simulink model "Simulation"  (R2018a)
settings: Solver=VariableStepAuto  StartTime=0.0  StopTime=inf  RelTol=1e-3
libraries: powerlib x28, simulink x3, rectifier_leg x3, inverter_leg x3, powerlib_meascontrol x1
settings Model: Creator=elasfory  LastModifiedBy=AL-MOSTAFA

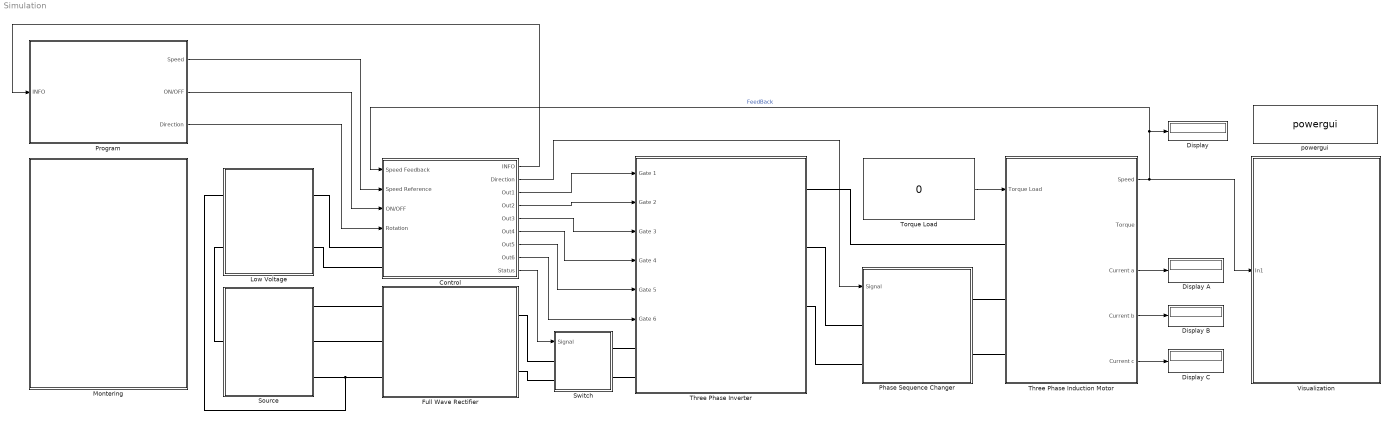
== system Simulation ==
  Control : Subsystem
  Display : Display
  Display A : Display
  Display B : Display
  Display C : Display
  Full Wave Rectifier : Subsystem
  Low Voltage : Subsystem
  Montering : Subsystem
  Phase Sequence Changer : Subsystem
  Program : Subsystem
  Source : Subsystem
  Switch : Subsystem
  Three Phase Induction Motor : Subsystem
  Three Phase Inverter : Subsystem
  Torque Load : Constant  Value=0
  Visualization : Subsystem
  powergui : powerlib/powergui  Priority=1  SimulationMode=Continuous  SampleTime=50e-6  frequency=60  Iterations=50  frequencyindice=0  Pbase=100e6  ErrMax=1e-4  UnitsV=kV  UnitsW=MW  buscounter=0  FunctionMessages=off  echomessages=off  EnableUseOfTLC=off  CurrentSourceSwitches=off  DisableSnubberDevices=off  DisableRonSwitches=off  DisableVfSwitches=off  DisplayEquations=off  SolverType=Tustin/Backward Euler (TBE)  Interpol=off  ExternalGateDelay=off  methode=off  Ts=100  x0status=blocks  SPID=on  SwTol=0  HookPort=off  RestoreLinks=warning  ResistiveCurrentMeasurement=off  Frange=[0:2:500]  Ylog=off  Xlog=on  ShowGrid=off  save=off  variable=ZData  structure=0  ZoomFFT=off  StartTime=0.0  cycles=1  DisplayStyle=1  fundamental=60  FreqAxis=off  MaxFrequency=1000  frequencyindicesteady=1  RmsSteady=1  display=off
  wires:
  Control/8(Out6) -> Three Phase Inverter/6(Gate 6)
  Control/7(Out5) -> Three Phase Inverter/5(Gate 5)
  Control/6(Out4) -> Three Phase Inverter/4(Gate 4)
  Control/5(Out3) -> Three Phase Inverter/3(Gate 3)
  Control/4(Out2) -> Three Phase Inverter/2(Gate 2)
  Control/3(Out1) -> Three Phase Inverter/1(Gate 1)
  Three Phase Induction Motor/1(Speed) -> Visualization/1(In1), Display/1, Control/1(Speed Feedback)  "FeedBack"
  Torque Load/1 -> Three Phase Induction Motor/1(Torque Load)
  Program/1(Speed) -> Control/2(Speed Reference)
  Three Phase Induction Motor/3(Current a) -> Display A/1
  Three Phase Induction Motor/4(Current b) -> Display B/1
  Three Phase Induction Motor/5(Current c) -> Display C/1
  Program/2(ON/OFF) -> Control/3(ON/OFF)
  Program/3(Direction) -> Control/4(Rotation)
  Control/9(Status) -> Switch/1(Signal)
  Control/2(Direction) -> Phase Sequence Changer/1(Signal)
  Control/1(INFO) -> Program/1(INFO)
  connections:
  Source/RConn1 -- Full Wave Rectifier/LConn1
  Source/RConn2 -- Full Wave Rectifier/LConn2
  Source/RConn3 -- Low Voltage/LConn1 -- Full Wave Rectifier/LConn3
  Three Phase Inverter/RConn1 -- Three Phase Induction Motor/LConn1
  Three Phase Inverter/RConn2 -- Phase Sequence Changer/LConn1
  Three Phase Inverter/RConn3 -- Phase Sequence Changer/LConn2
  Phase Sequence Changer/RConn1 -- Three Phase Induction Motor/LConn2
  Phase Sequence Changer/RConn2 -- Three Phase Induction Motor/LConn3
  Full Wave Rectifier/RConn1 -- Switch/LConn1
  Full Wave Rectifier/RConn2 -- Switch/LConn2
  Switch/RConn1 -- Three Phase Inverter/LConn1
  Switch/RConn2 -- Three Phase Inverter/LConn2
  Low Voltage/RConn1 -- Control/LConn1
  Low Voltage/RConn2 -- Control/LConn2
  Source/LConn1 -- Low Voltage/LConn2

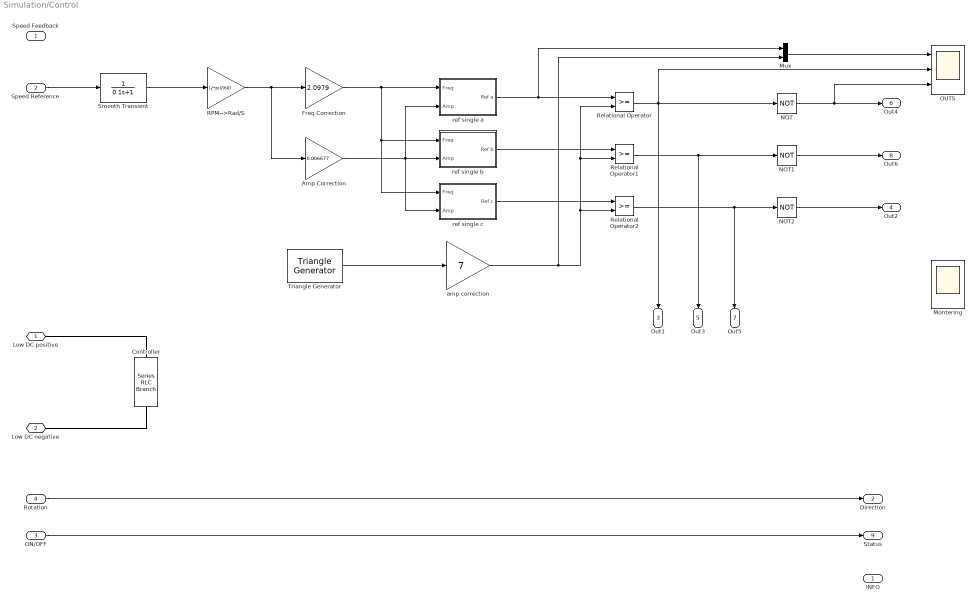
== system Simulation/Control ==
  Speed Feedback : Inport
  Speed Reference : Inport  Port=2
  ON/OFF : Inport  Port=3
  Rotation : Inport  Port=4
  Amp Correction : Gain  Gain=0.006677
  Controller : powerlib/Elements/Series RLC Branch  LConnTagsString=__new0  RConnTagsString=__new0  BranchType=R  Resistance=220  Inductance=1e-3  SetiL0=off  InitialCurrent=0  Capacitance=500*10^-6  Setx0=off  InitialVoltage=0  Measurements=None
  Freq Correction : Gain  Gain=2.0979
  Montering : Scope  NumInputPorts=2
  Mux : Mux  Inputs=2
  NOT : Logic  Operator=NOT  IconShape=distinctive  AllPortsSameDT=off  OutDataTypeStr=boolean
  NOT1 : Logic  Operator=NOT  IconShape=distinctive  AllPortsSameDT=off  OutDataTypeStr=boolean
  NOT2 : Logic  Operator=NOT  IconShape=distinctive  AllPortsSameDT=off  OutDataTypeStr=boolean
  OUTS : Scope  NumInputPorts=3
  RPM-->Rad/S : Gain  Gain=(2*pi)/(60)
  Relational Operator : RelationalOperator  OutDataTypeStr=boolean  RndMeth=Simplest
  Relational Operator1 : RelationalOperator  OutDataTypeStr=boolean  RndMeth=Simplest
  Relational Operator2 : RelationalOperator  OutDataTypeStr=boolean  RndMeth=Simplest
  Smooth Transient : TransferFcn  Denominator=[0.1 1]
  Triangle Generator : powerlib_meascontrol/Pulse & Signal Generators/Triangle Generator  Freq=1e3  Phase=90  Ts=0
  amp correction : Gain  Gain=7
  ref single a : Subsystem
  ref single b : Subsystem
  ref single c : Subsystem
  Low DC positive : PMIOPort  Side=Left
  Low DC negative : PMIOPort  Port=2  Side=Left
  INFO : Outport
  Direction : Outport  Port=2
  Out1 : Outport  Port=3
  Out2 : Outport  Port=4
  Out3 : Outport  Port=5
  Out4 : Outport  Port=6
  Out5 : Outport  Port=7
  Out6 : Outport  Port=8
  Status : Outport  Port=9
  wires:
  amp correction/1 -> Relational Operator/2, Relational Operator1/2, Relational Operator2/2, Mux/2
  ON/OFF/1 -> Status/1
  Rotation/1 -> Direction/1
  ref single a/1(Ref a) -> Mux/1, Relational Operator/1
  RPM-->Rad/S/1 -> Freq Correction/1, Amp Correction/1
  Freq Correction/1 -> ref single c/1(Freq), ref single b/1(Freq), ref single a/1(Freq)
  Amp Correction/1 -> ref single c/2(Amp), ref single a/2(Amp), ref single b/2(Amp)
  ref single b/1(Ref b) -> Relational Operator1/1
  ref single c/1(Ref c) -> Relational Operator2/1
  Relational Operator/1 -> OUTS/2, NOT/1, Out1/1
  Relational Operator1/1 -> NOT1/1, Out3/1
  Relational Operator2/1 -> NOT2/1, Out5/1
  NOT2/1 -> Out2/1
  NOT1/1 -> Out6/1
  NOT/1 -> Out4/1, OUTS/3
  Triangle Generator/1 -> amp correction/1
  Mux/1 -> OUTS/1
  Speed Reference/1 -> Smooth Transient/1
  Smooth Transient/1 -> RPM-->Rad/S/1
  connections:
  Controller/LConn1 -- Low DC positive/RConn1
  Low DC negative/RConn1 -- Controller/RConn1

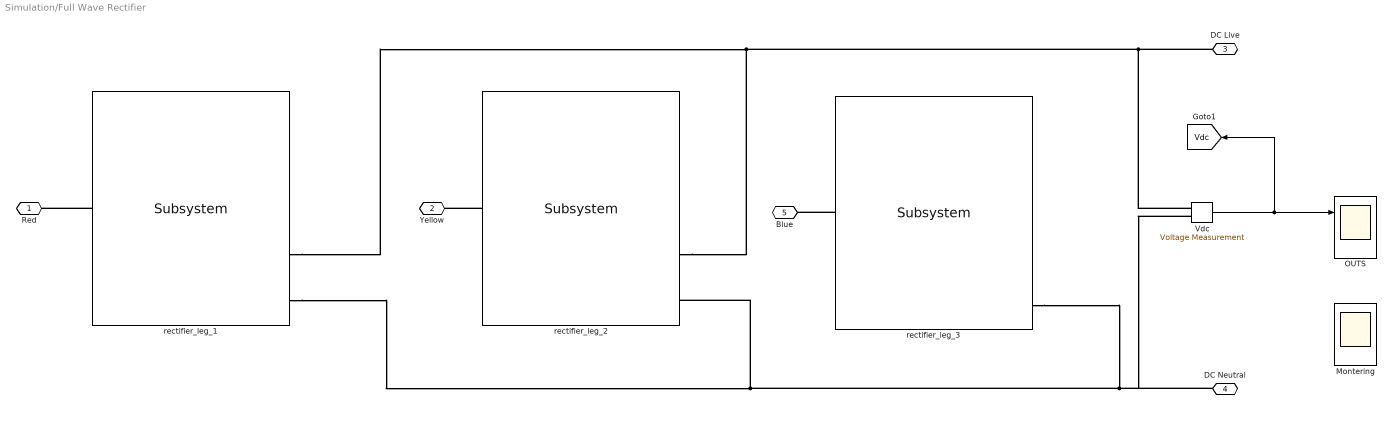
== system Simulation/Full Wave Rectifier ==
  Montering : Scope  NumInputPorts=4
  OUTS : Scope  NumInputPorts=2
  Vdc : powerlib/Measurements/Voltage Measurement  PhasorSimulation=off  OutputType=Complex  PSBequivalent=0
  rectifier_leg_1 : rectifier_leg/Subsystem
  rectifier_leg_2 : rectifier_leg/Subsystem
  rectifier_leg_3 : rectifier_leg/Subsystem
  Red : PMIOPort  Side=Left
  Yellow : PMIOPort  Port=2  Side=Left
  DC Live : PMIOPort  Port=3  Side=Right
  DC Neutral : PMIOPort  Port=4  Side=Right
  Blue : PMIOPort  Port=5  Side=Left
  tag scope: Vdc=global
  wires:
  Vdc/1 -> OUTS/1, [Vdc]
  connections:
  DC Live/RConn1 -- Vdc/LConn1 -- rectifier_leg_1/RConn1 -- rectifier_leg_2/RConn1
  rectifier_leg_1/LConn1 -- Red/RConn1
  rectifier_leg_2/LConn1 -- Yellow/RConn1
  rectifier_leg_3/LConn1 -- Blue/RConn1
  rectifier_leg_3/RConn2 -- DC Neutral/RConn1 -- Vdc/LConn2 -- rectifier_leg_2/RConn2 -- rectifier_leg_1/RConn2

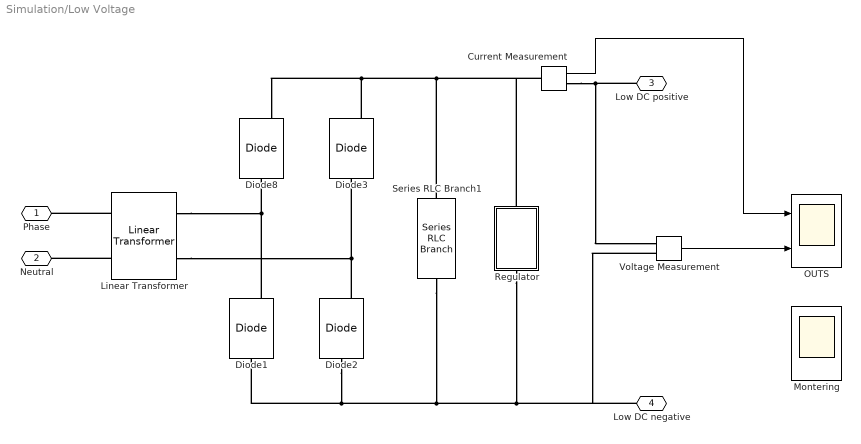
== system Simulation/Low Voltage ==
  Current Measurement : powerlib/Measurements/Current Measurement  PhasorSimulation=off  OutputType=Complex  PSBequivalent=0
  Diode{1..3,8} (4 alike) : powerlib/Power Electronics/Diode  Ron=0.001  Lon=0  Vf=0.8  IC=0  UseSnubber=0  Rs=500  Cs=250e-9  Measurements=on
  Linear Transformer : powerlib/Elements/Linear Transformer  UNITS=pu  NominalPower=[ 1000 50 ]  winding1=[380 0.002 0.08]  winding2=[8.25 0.002 0.08]  ThreeWindings=off  winding3=[3.15e+05 0.002 0.08]  RmLm=[500.02 500]  Measurements=None  DataType=off
  Montering : Scope  NumInputPorts=4
  OUTS : Scope  NumInputPorts=2
  Regulator : Subsystem
  Series RLC Branch1 : powerlib/Elements/Series RLC Branch  LConnTagsString=__new0  RConnTagsString=__new0  BranchType=RC  Resistance=0.1  Inductance=1e-3  SetiL0=off  InitialCurrent=0  Capacitance=500*10^-6  Setx0=off  InitialVoltage=0  Measurements=None
  Voltage Measurement : powerlib/Measurements/Voltage Measurement  PhasorSimulation=off  OutputType=Complex  PSBequivalent=0
  Phase : PMIOPort  Side=Left
  Neutral : PMIOPort  Port=2  Side=Left
  Low DC positive : PMIOPort  Port=3  Side=Right
  Low DC negative : PMIOPort  Port=4  Side=Right
  wires:
  Voltage Measurement/1 -> OUTS/2
  Current Measurement/1 -> OUTS/1
  connections:
  Linear Transformer/LConn1 -- Phase/RConn1
  Linear Transformer/LConn2 -- Neutral/RConn1
  Diode1/RConn1 -- Linear Transformer/RConn1 -- Diode8/LConn1
  Diode2/RConn1 -- Linear Transformer/RConn2 -- Diode3/LConn1
  Diode3/RConn1 -- Current Measurement/LConn1 -- Regulator/RConn1 -- Series RLC Branch1/LConn1 -- Diode8/RConn1
  Diode2/LConn1 -- Regulator/LConn1 -- Voltage Measurement/LConn2 -- Low DC negative/RConn1 -- Series RLC Branch1/RConn1 -- Diode1/LConn1
  Low DC positive/RConn1 -- Current Measurement/RConn1 -- Voltage Measurement/LConn1

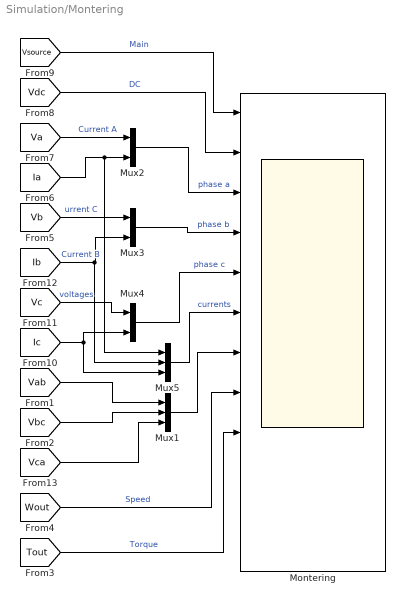
== system Simulation/Montering ==
  Montering : Scope  NumInputPorts=12
  Mux1 : Mux  Inputs=3
  Mux2 : Mux  Inputs=2
  Mux3 : Mux  Inputs=2
  Mux4 : Mux  Inputs=2
  Mux5 : Mux  Inputs=3
  wires:
  Mux5/1 -> Montering/6  "currents"
  [Vc] -> Mux4/1  "voltages"
  [Tout] -> Montering/9  "Torque"
  [Wout] -> Montering/8  "Speed"
  [Ic] -> Mux5/3, Mux4/2
  [Vdc] -> Montering/2  "DC"
  [Vb] -> Mux3/1  "urrent C"
  [Vbc] -> Mux1/2
  Mux1/1 -> Montering/7
  [Va] -> Mux2/1  "Current A"
  [Ib] -> Mux5/2, Mux3/2
  [Vca] -> Mux1/3
  [Vab] -> Mux1/1
  Mux3/1 -> Montering/4  "phase b"
  Mux2/1 -> Montering/3  "phase a"
  Mux4/1 -> Montering/5  "phase c"
  [Ia] -> Mux5/1, Mux2/2  "Current B"
  [Vsource] -> Montering/1  "Main"

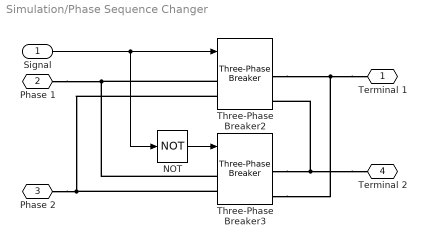
== system Simulation/Phase Sequence Changer ==
  Signal : Inport
  NOT : Logic  Operator=NOT  IconShape=distinctive  AllPortsSameDT=off  OutDataTypeStr=boolean
  Three-Phase Breaker2 : powerlib/Elements/Three-Phase Breaker  InitialState=closed  SwitchA=on  SwitchB=on  SwitchC=on  SwitchTimes="[1/60  5/60]"  External=on  BreakerResistance=0.01  SnubberResistance=10^6  SnubberCapacitance=inf  Measurements=Breaker currents
  Three-Phase Breaker3 : powerlib/Elements/Three-Phase Breaker  InitialState=open  SwitchA=on  SwitchB=on  SwitchC=on  SwitchTimes="[1/60  5/60]"  External=on  BreakerResistance=0.01  SnubberResistance=10^6  SnubberCapacitance=inf  Measurements=Breaker currents
  Terminal 1 : PMIOPort  Side=Right
  Phase 1 : PMIOPort  Port=2  Side=Left
  Phase 2 : PMIOPort  Port=3  Side=Left
  Terminal 2 : PMIOPort  Port=4  Side=Right
  wires:
  NOT/1 -> Three-Phase Breaker3/1
  Signal/1 -> Three-Phase Breaker2/1, NOT/1
  connections:
  Phase 1/RConn1 -- Three-Phase Breaker2/LConn2 -- Three-Phase Breaker3/LConn2
  Phase 2/RConn1 -- Three-Phase Breaker3/LConn3 -- Three-Phase Breaker2/LConn3
  Terminal 1/RConn1 -- Three-Phase Breaker3/RConn3 -- Three-Phase Breaker2/RConn2
  Terminal 2/RConn1 -- Three-Phase Breaker3/RConn2 -- Three-Phase Breaker2/RConn3

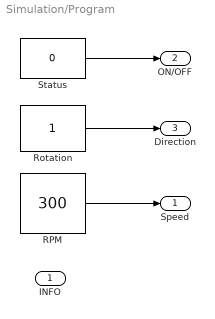
== system Simulation/Program ==
  INFO : Inport
  RPM : Constant  Value=300
  Rotation : Constant
  Status : Constant  Value=0
  Speed : Outport
  ON/OFF : Outport  Port=2
  Direction : Outport  Port=3
  wires:
  RPM/1 -> Speed/1
  Rotation/1 -> Direction/1
  Status/1 -> ON/OFF/1

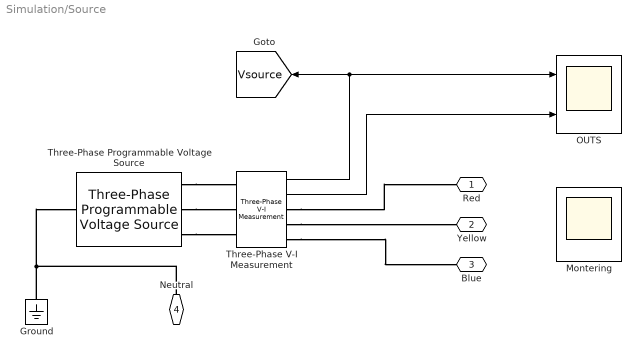
== system Simulation/Source ==
  Ground : powerlib/Elements/Ground  LConnTagsString=a
  Montering : Scope  NumInputPorts=4
  OUTS : Scope  NumInputPorts=2
  Three-Phase Programmable Voltage Source : powerlib/Electrical Sources/Three-Phase Programmable Voltage Source  PositiveSequence="[380  0 50]"  VariationEntity=None  VariationType=Table of time-amplitude pairs  VariationTypeAlt=Step  VariationStep=0.5  VariationRate=10  VariationMagnitude=0.3  VariationFrequency=2  VariationTiming=[1 2]  VariationPhaseA=off  Amplitudes=[1 0.8 1.2 1.0]  TimeValues=[0 0.1 0.15 0.2]  HarmonicGeneration=off  HarmonicA=[3 0.2 -25 0]  HarmonicB=[2 0.15 35 2]  Timing="[0.05  3]"  BusType=swing  Pref=0  Qref=0  Qmin=-inf  Qmax=inf
  Three-Phase V-I Measurement : powerlib/Measurements/Three-Phase V-I Measurement  VoltageMeasurement=phase-to-ground  SetLabelV=off  LabelV=Vabc  Vpu=off  VpuLL=off  CurrentMeasurement=yes  SetLabelI=off  LabelI=Iabc  Ipu=off  Pbase=100e6  Vbase=500e3  OutputType=Complex  PhasorSimulation=off  PSBequivalent=0
  Red : PMIOPort  Side=Right
  Yellow : PMIOPort  Port=2  Side=Right
  Blue : PMIOPort  Port=3  Side=Right
  Neutral : PMIOPort  Port=4  Side=Left
  tag scope: Vsource=global
  wires:
  Three-Phase V-I Measurement/1 -> [Vsource], OUTS/1
  Three-Phase V-I Measurement/2 -> OUTS/2
  connections:
  Three-Phase V-I Measurement/RConn3 -- Blue/RConn1
  Three-Phase V-I Measurement/RConn1 -- Red/RConn1
  Three-Phase V-I Measurement/RConn2 -- Yellow/RConn1
  Three-Phase Programmable Voltage Source/RConn1 -- Three-Phase V-I Measurement/LConn1
  Three-Phase Programmable Voltage Source/RConn2 -- Three-Phase V-I Measurement/LConn2
  Three-Phase Programmable Voltage Source/RConn3 -- Three-Phase V-I Measurement/LConn3
  Ground/LConn1 -- Three-Phase Programmable Voltage Source/LConn1 -- Neutral/RConn1

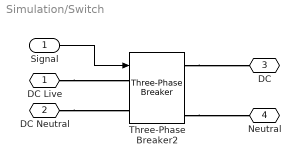
== system Simulation/Switch ==
  Signal : Inport
  Three-Phase Breaker2 : powerlib/Elements/Three-Phase Breaker  InitialState=closed  SwitchA=on  SwitchB=on  SwitchC=on  SwitchTimes="[1/60  5/60]"  External=on  BreakerResistance=0.01  SnubberResistance=10^6  SnubberCapacitance=inf  Measurements=Breaker currents
  DC Live : PMIOPort  Side=Left
  DC Neutral : PMIOPort  Port=2  Side=Left
  DC : PMIOPort  Port=3  Side=Right
  Neutral : PMIOPort  Port=4  Side=Right
  wires:
  Signal/1 -> Three-Phase Breaker2/1
  connections:
  Three-Phase Breaker2/RConn3 -- Neutral/RConn1
  DC Neutral/RConn1 -- Three-Phase Breaker2/LConn3
  Three-Phase Breaker2/RConn1 -- DC/RConn1
  DC Live/RConn1 -- Three-Phase Breaker2/LConn1

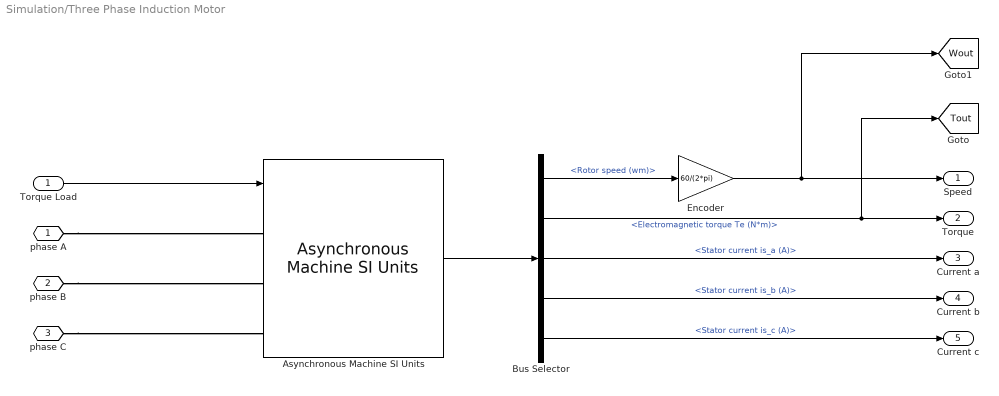
== system Simulation/Three Phase Induction Motor ==
  Torque Load : Inport
  Asynchronous Machine SI Units : powerlib/Machines/Asynchronous Machine SI Units  RotorType=Squirrel-cage  PresetModel="15:  5.4 HP (4KW)   400 V  50Hz 1430 RPM"  MechanicalLoad=Torque Tm  ShowDetailedParameters=on  ReferenceFrame=Stationary  Units=SI  MeasurementBus=off  NominalParameters=[4000 400 50]  Stator=[1.405 0.005839]  Rotor=[1.395 0.005839]  Cage1=[0.4155 0.002066]  Cage2=[0.4168 0.0003495]  Lm=0.1722  Mechanical=[0.0131 0.002985 2]  PolePairs=2  InitialConditions=[1 0 0 0 0 0 0 0]  SimulateSaturation=off  Saturation=[14.03593122, 27.81365428, 53.79336849, 72.68890987, 97.98006896, 148.6815601, 215.7428561, 302.9841135, 428.7778367 ; 230, 322, 414, 460, 506, 552, 598, 644, 690]  LoadFlowParameters=1492000  TsPowergui=0  TsBlock=-1  IterativeModel=Trapezoidal non iterative  IterativeDiscreteModel=Trapezoidal non iterative  Pmec=1.492e+006
  Bus Selector : BusSelector  OutputSignals=Mechanical.Rotor speed (wm),Mechanical.Electromagnetic torque Te (N*m),Stator measurements.Stator current is_a (A),Stator measurements.Stator current is_b (A),Stator measurements.Stator current is_c (A)
  Encoder : Gain  Gain=60/(2*pi)
  phase A : PMIOPort  Side=Left
  phase B : PMIOPort  Port=2  Side=Left
  phase C : PMIOPort  Port=3  Side=Left
  Speed : Outport
  Torque : Outport  Port=2
  Current a : Outport  Port=3
  Current b : Outport  Port=4
  Current c : Outport  Port=5
  tag scope: Tout=global, Wout=global
  wires:
  Asynchronous Machine SI Units/1 -> Bus Selector/1
  Bus Selector/2 -> [Tout], Torque/1  "<Electromagnetic torque Te (N*m)>"
  Torque Load/1 -> Asynchronous Machine SI Units/1
  Bus Selector/3 -> Current a/1  "<Stator current is_a (A)>"
  Bus Selector/4 -> Current b/1  "<Stator current is_b (A)>"
  Bus Selector/5 -> Current c/1  "<Stator current is_c (A)>"
  Bus Selector/1 -> Encoder/1  "<Rotor speed (wm)>"
  Encoder/1 -> Speed/1, [Wout]
  connections:
  phase B/RConn1 -- Asynchronous Machine SI Units/LConn2
  phase A/RConn1 -- Asynchronous Machine SI Units/LConn1
  phase C/RConn1 -- Asynchronous Machine SI Units/LConn3

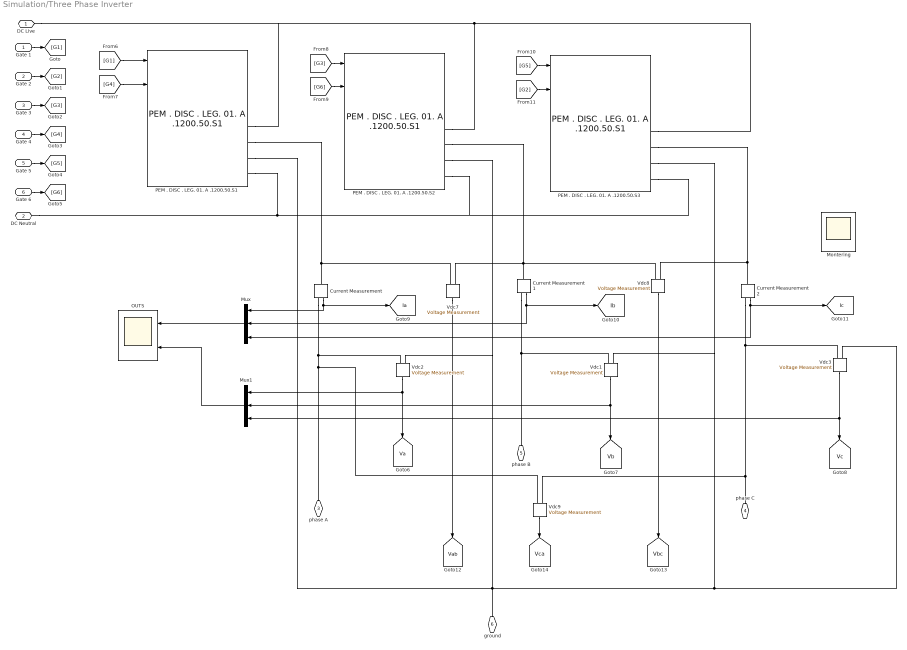
== system Simulation/Three Phase Inverter ==
  Gate 1 : Inport
  Gate 2 : Inport  Port=2
  Gate 3 : Inport  Port=3
  Gate 4 : Inport  Port=4
  Gate 5 : Inport  Port=5
  Gate 6 : Inport  Port=6
  Current Measurement : powerlib/Measurements/Current Measurement  PhasorSimulation=off  OutputType=Complex  PSBequivalent=0
  Current Measurement1 : powerlib/Measurements/Current Measurement  PhasorSimulation=off  OutputType=Complex  PSBequivalent=0
  Current Measurement2 : powerlib/Measurements/Current Measurement  PhasorSimulation=off  OutputType=Complex  PSBequivalent=0
  Montering : Scope  NumInputPorts=4
  Mux : Mux  Inputs=3
  Mux1 : Mux  Inputs=3
  OUTS : Scope  NumInputPorts=2
  PEM . DISC . LEG. 01. A .1200.50.S1 : inverter_leg/PEM . DISC . LEG. 01. A .1200.50.S1
  PEM . DISC . LEG. 01. A .1200.50.S2 : inverter_leg/PEM . DISC . LEG. 01. A .1200.50.S1
  PEM . DISC . LEG. 01. A .1200.50.S3 : inverter_leg/PEM . DISC . LEG. 01. A .1200.50.S1
  Vdc{1..3,7..9} (6 alike) : powerlib/Measurements/Voltage Measurement  PhasorSimulation=off  OutputType=Complex  PSBequivalent=0
  DC Live : PMIOPort  Side=Left
  DC Neutral : PMIOPort  Port=2  Side=Left
  phase A : PMIOPort  Port=3  Side=Right
  phase C : PMIOPort  Port=4  Side=Right
  phase B : PMIOPort  Port=5  Side=Right
  ground : PMIOPort  Port=6  Side=Right
  tag scope: Ia=global, Ib=global, Ic=global, Va=global, Vab=global, Vb=global, Vbc=global, Vc=global, Vca=global
  wires:
  Gate 1/1 -> [G1]
  Gate 2/1 -> [G2]
  Gate 3/1 -> [G3]
  Gate 4/1 -> [G4]
  Gate 5/1 -> [G5]
  Gate 6/1 -> [G6]
  [G4] -> PEM . DISC . LEG. 01. A .1200.50.S1/2
  [G1] -> PEM . DISC . LEG. 01. A .1200.50.S1/1
  [G6] -> PEM . DISC . LEG. 01. A .1200.50.S2/2
  [G3] -> PEM . DISC . LEG. 01. A .1200.50.S2/1
  [G5] -> PEM . DISC . LEG. 01. A .1200.50.S3/1
  [G2] -> PEM . DISC . LEG. 01. A .1200.50.S3/2
  Current Measurement/1 -> [Ia], Mux/1
  Current Measurement1/1 -> Mux/2, [Ib]
  Current Measurement2/1 -> Mux/3, [Ic]
  Vdc2/1 -> [Va], Mux1/1
  Vdc1/1 -> Mux1/2, [Vb]
  Vdc3/1 -> Mux1/3, [Vc]
  Vdc9/1 -> [Vca]
  Vdc7/1 -> [Vab]
  Vdc8/1 -> [Vbc]
  Mux/1 -> OUTS/1
  Mux1/1 -> OUTS/2
  connections:
  PEM . DISC . LEG. 01. A .1200.50.S1/RConn1 -- DC Live/RConn1 -- PEM . DISC . LEG. 01. A .1200.50.S3/RConn1 -- PEM . DISC . LEG. 01. A .1200.50.S2/RConn1
  PEM . DISC . LEG. 01. A .1200.50.S3/RConn4 -- PEM . DISC . LEG. 01. A .1200.50.S2/RConn4 -- PEM . DISC . LEG. 01. A .1200.50.S1/RConn4 -- DC Neutral/RConn1
  ground/RConn1 -- PEM . DISC . LEG. 01. A .1200.50.S1/RConn3 -- PEM . DISC . LEG. 01. A .1200.50.S3/RConn3 -- Vdc1/LConn2 -- Vdc3/LConn2 -- PEM . DISC . LEG. 01. A .1200.50.S2/RConn3 -- Vdc2/LConn2
  Current Measurement/LConn1 -- PEM . DISC . LEG. 01. A .1200.50.S1/RConn2 -- Vdc7/LConn1
  Current Measurement/RConn1 -- Vdc2/LConn1 -- Vdc9/LConn2 -- phase A/RConn1
  Current Measurement1/RConn1 -- Vdc1/LConn1 -- phase B/RConn1
  Current Measurement1/LConn1 -- PEM . DISC . LEG. 01. A .1200.50.S2/RConn2 -- Vdc8/LConn1 -- Vdc7/LConn2
  Current Measurement2/RConn1 -- Vdc3/LConn1 -- Vdc9/LConn1 -- phase C/RConn1
  Current Measurement2/LConn1 -- PEM . DISC . LEG. 01. A .1200.50.S3/RConn2 -- Vdc8/LConn2

== system Simulation/Visualization ==
  In1 : Inport
  Angluar_Velocity : ToWorkspace  VariableName=Speed  SaveFormat=Timeseries  SampleTime=1/60
  wires:
  In1/1 -> Angluar_Velocity/1

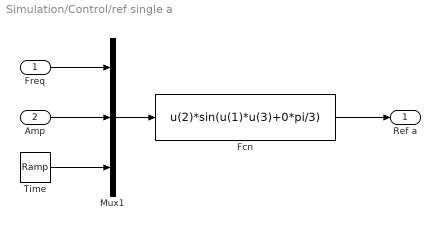
== system Simulation/Control/ref single a ==
  Freq : Inport
  Amp : Inport  Port=2
  Fcn : Fcn  Expr=u(2)*sin(u(1)*u(3)+0*pi/3)
  Mux1 : Mux  Inputs=3
  Time : simulink/Sources/Ramp  slope=1  start=0  InitialOutput=0
  Ref a : Outport
  wires:
  Mux1/1 -> Fcn/1
  Fcn/1 -> Ref a/1
  Freq/1 -> Mux1/1
  Time/1 -> Mux1/3
  Amp/1 -> Mux1/2

== system Simulation/Control/ref single b ==
  Freq : Inport
  Amp : Inport  Port=2
  Fcn : Fcn  Expr=u(2)*sin(u(1)*u(3)-2*pi/3)
  Mux1 : Mux  Inputs=3
  Time : simulink/Sources/Ramp  slope=1  start=0  InitialOutput=0
  Ref b : Outport
  wires:
  Amp/1 -> Mux1/2
  Time/1 -> Mux1/3
  Fcn/1 -> Ref b/1
  Mux1/1 -> Fcn/1
  Freq/1 -> Mux1/1

== system Simulation/Control/ref single c ==
  Freq : Inport
  Amp : Inport  Port=2
  Fcn : Fcn  Expr=u(2)*sin(u(1)*u(3)+2*pi/3)
  Mux1 : Mux  Inputs=3
  Time : simulink/Sources/Ramp  slope=1  start=0  InitialOutput=0
  Ref c : Outport
  wires:
  Amp/1 -> Mux1/2
  Time/1 -> Mux1/3
  Fcn/1 -> Ref c/1
  Mux1/1 -> Fcn/1
  Freq/1 -> Mux1/1

== system Simulation/Low Voltage/Regulator ==
  DC Voltage Source : powerlib/Electrical Sources/DC Voltage Source  Amplitude=5  Measurements=None
  -VE : PMIOPort  Side=Left
  +VE : PMIOPort  Port=2  Side=Right
  connections:
  DC Voltage Source/RConn1 -- +VE/RConn1
  DC Voltage Source/LConn1 -- -VE/RConn1
